simulink model "PID"  (R2021b)
settings: Solver=VariableStepAuto  StartTime=0.0  StopTime=10.0  RelTol=1e-3
values from neighbouring files (symbols this model uses):
  hd = 2    [OneDOF.m]    (also in PID_Controller.m = 100)
  hi = 10    [OneDOF.m]    (also in PID_Controller.m = 3)
  hp = 0.01    [OneDOF.m]    (also in PID_Controller.m = 0.001)
settings Model: Creator=thomasperrein  LastModifiedBy=thomasperrein

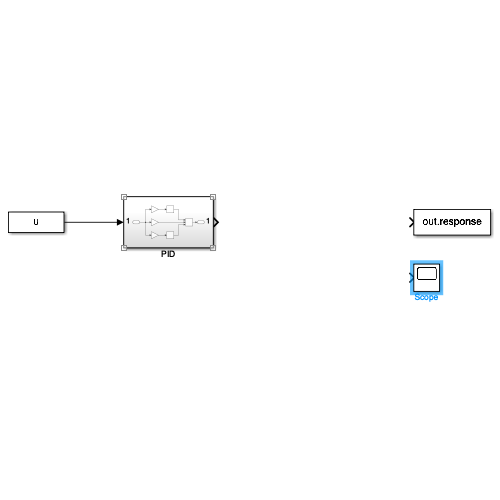
[thumbnail: Simulink's stored preview of the top-level diagram]
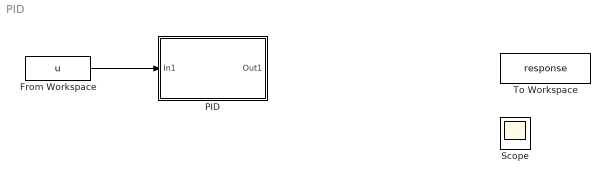
== system PID ==
  From Workspace : FromWorkspace  VariableName=u
  PID : Subsystem
  Scope : Scope
  To Workspace : ToWorkspace  VariableName=response  SaveFormat=Timeseries  SampleTime=-1
  wires:
  From Workspace/1 -> PID/1(In1)

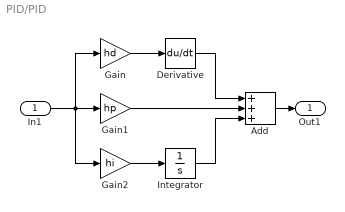
== system PID/PID ==
  In1 : Inport
  Add : Sum  Inputs=+++
  Derivative : Derivative
  Gain : Gain  Gain=hd
  Gain1 : Gain  Gain=hp
  Gain2 : Gain  Gain=hi
  Integrator : Integrator
  Out1 : Outport
  wires:
  Add/1 -> Out1/1
  Gain2/1 -> Integrator/1
  Gain1/1 -> Add/2
  Derivative/1 -> Add/1
  In1/1 -> Gain/1, Gain2/1, Gain1/1
  Gain/1 -> Derivative/1
  Integrator/1 -> Add/3
